simulink library "neuromorphic_blocks"  (R2022a)
settings: Solver=VariableStepAuto  StartTime=0.0  StopTime=10.0  RelTol=1e-3
libraries: $bdroot x31, simulink x7
(part 1 of 2)
settings Model: Creator=chris  LastModifiedBy=chris

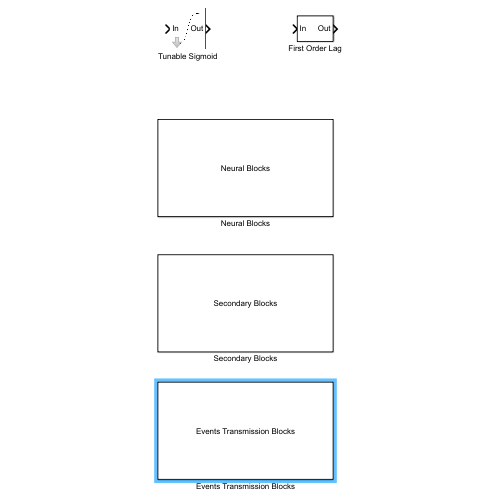
[thumbnail: Simulink's stored preview of the top-level diagram]
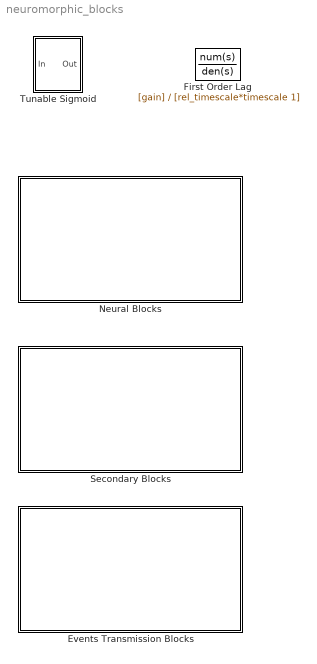
== system neuromorphic_blocks ==
  Events Transmission Blocks : Subsystem
      mask Display: disp('Events Transmission Blocks');
  First Order Lag : TransferFcn  Numerator=[gain]  Denominator=[rel_timescale*timescale 1]  mask(First Order Lag){gain=1, timescale=0.004, rel_timescale=1}
      mask help: Wrapper around Low-Pass Filter block of simulink to make it consistent with other blocks in the toolbox.
      mask DialogControl gain_text Prompt: Gain
      mask DialogControl timescale_text Prompt: Timescale
      mask DialogControl rel_timescale_text Prompt: Relative Timescale
      mask Display:
      | port_label('output', 1, 'Out');
      | port_label('input', 1, 'In');
  Neural Blocks : Subsystem
      mask Display: disp('Neural Blocks');
  Secondary Blocks : Subsystem
      mask Display: disp('Secondary Blocks');
  Tunable Sigmoid : Subsystem  mask(Tunable Sigmoid){nonlinearity_type=Sigmoid, gain_source=Internal, gain=0, bias=0, slope=1}
      mask prompts: gain_source "Source"; gain "Value"; bias "Value"; slope "Value"
      mask help:
      | Sigmoid where gain can be set by external input.
      | The block can be set in Tanh or Sigmoid mode.
      mask init:
      | mask  = Simulink.Mask.get(gcb);
      | 
      |     %type_chosen = mask.getParameter('nonlinearity_type').Value;
      |     %set_param([gcb '/VSNK' ],'LabelModeActiveChoice', type_chosen);
      |     %set_param([gcb '/VSRC' ],'LabelModeActiveChoice', type_chosen);
      |     %disp(type_chosen)
      | 
      |     switch mask.getParameter('nonlinearity_type').Value
      |         case 'Sigmoid'
      |             set_param([gcb '/VSNK' ],'LabelModeActiveChoice', 'Sigmoid');
      |             set_param([gcb '/VSRC' ],'LabelModeActiveChoice', 'Sigmoid');
      |         case 'Tanh'
      |             set_param([gcb '/VSNK' ],'LabelModeActiveChoice', 'Tanh');
      |             set_param([gcb '/VSRC' ],'LabelModeActiveChoice', 'Tanh');
      |     end
      | 
      | 
      |     type = {get_param([gcb '/gain'],'BlockType')};
      |     switch mask.getParameter('gain_source').Value
      |         case 'Internal'
      |             if ismember(type, {'Inport'})
      |                 replace_block([gcb '/gain'], 'Inport', 'Constant', 'noprompt');
      |             end
      |             set_param([gcb '/gain'],'Value','gain');
      |         case 'External'
      |             if ismember(type, {'Constant'})
      |                 replace_block([gcb '/gain'], 'Constant', 'Inport', 'noprompt');
      |             end
      |     end
      mask TypeOptions nonlinearity_type: Sigmoid | Tanh
      mask TypeOptions gain_source: Internal | External
      mask Callback gain_source:
      | mask  = Simulink.Mask.get(gcb);
      |     switch mask.getParameter('gain_source').Value
      |         case 'Internal'
      |             mask.getParameter('gain').Enabled = 'on';
      |         case 'External'
      |             mask.getParameter('gain').Enabled = 'off';
      |     end
      mask DialogControl type_text Prompt: Type
      mask DialogControl gain_text Prompt: Gain
      mask DialogControl bias_text Prompt: Bias
      mask DialogControl slope_text Prompt: Slope
      mask Display:
      | mask  = Simulink.Mask.get(gcb);
      | [gain, gain_converted] = str2num(mask.getParameter('gain').Value);
      | [slope, slope_converted] = str2num(mask.getParameter('slope').Value);
      | 
      | if strcmp(mask.getParameter('gain_source').Value,'Internal') ...
      |    && gain_converted && slope_converted && gain*slope < 0
      |     image('icons/tanh_reversed.jpg');
      | else
      |     image('icons/tanh.jpg');
      | end
      | 
      | 
      | port_label('output', 1, 'Out');
      | 
      | simBlockH = get_param(gcb, 'Handle');
      | portH = find_system(simBlockH, 'LookUnderMasks', 'on', 'FollowLinks', 'on', 'SearchDepth', 1, 'BlockType', 'Inport');
      | portNames = cellstr(get_param(portH, 'Name'));
      | portNum = cellstr(get_param(portH, 'Port'));
      | for i = 1:length(portNames)
      |     if ~isempty(portNames{i})
      |         num = str2num(['uint8(' portNum{i} ')']);
      |         port_label('input', num, portNames{i});
      |     end
      | end

== system neuromorphic_blocks/Events Transmission Blocks ==
  Continuous to Event : Subsystem  mask(Continuous to Event){thresh=0}
      mask prompts: thresh "Value"
      mask DialogControl thresh_text Prompt: Threshold
      mask Display:
      | port_label('output', 1, 'Out');
      | port_label('input', 1, 'In');
  Event Loss : Subsystem  mask(Event Loss){loss_prob=0, seed=-1, seed_mem=randi([0, 100000])}
      mask prompts: loss_prob "Value"; seed "Value"
      mask init:
      | mask  = Simulink.Mask.get(gcb);
      |     switch mask.getParameter('seed').Value
      |         case '-1'
      |             mask.getParameter('seed_mem').Value = 'randi([0, 100000])';
      |         otherwise
      |             mask.getParameter('seed_mem').Value = mask.getParameter('seed').Value;
      |     end
      mask DialogControl loss_prob_text Prompt: Probability of lost event
      mask DialogControl seed_text Prompt: Seed (-1 for random seed)
      mask Display:
      | port_label('output', 1, 'Out');
      | port_label('input', 1, 'In');
  Event to Continuous : Subsystem  mask(Event to Continuous){gain=0}
      mask prompts: gain "Value"
      mask DialogControl gain_text Prompt: Event gain
      mask Display:
      | port_label('output', 1, 'Out');
      | port_label('input', 1, 'In');
  Event to Fixed Width Pulse : Subsystem  mask(Event to Fixed Width Pulse){pulse_width=0}
      mask prompts: pulse_width "Value"
      mask DialogControl pulse_width_text Prompt: Pulse Width
      mask Display:
      | port_label('output', 1, 'Out');
      | port_label('input', 1, 'In');

== system neuromorphic_blocks/Neural Blocks ==
  Modulatory Synapse : Subsystem  mask(Modulatory Synapse){base_val=0, gsyn_pos_source=Internal, gsyn_pos=0, gsyn_neg_source=Internal, gsyn_neg=0, timescale=0.004, rel_timescale=1000, input=Events, dsyn_pos=0, dsyn_neg=0, msyn_pos=1, msyn_neg=1}
      mask prompts: base_val "Value"; gsyn_pos_source "Source"; gsyn_pos "Value"; gsyn_neg_source "Source"; gsyn_neg "Value"; timescale "Value"; rel_timescale "Value"; dsyn_pos "Value"; dsyn_neg "Value"; msyn_pos "Value"; msyn_neg "Value"
      mask init:
      | mask  = Simulink.Mask.get(gcb);
      | 
      |     switch mask.getParameter('input').Value
      |         case 'Events'
      |             set_param([gcb '/VSNK_pos'],'LabelModeActiveChoice', 'Events');
      |             set_param([gcb '/VSRC_pos'],'LabelModeActiveChoice', 'Events');
      |             set_param([gcb '/VSNK_neg'],'LabelModeActiveChoice', 'Events');
      |             set_param([gcb '/VSRC_neg'],'LabelModeActiveChoice', 'Events');
      |             %mask.getPortConstraint('in_main_type').Rule.DataType = {'boolean'};
      |             try
      |                 set_param([gcb '/V+'], 'Name', 'Ev+');
      |                 set_param([gcb '/V-'], 'Name', 'Ev-');
      |             catch E
      |             end
      |         case 'Voltage'
      |             set_param([gcb '/VSNK_pos'],'LabelModeActiveChoice', 'Voltage');
      |             set_param([gcb '/VSRC_pos'],'LabelModeActiveChoice', 'Voltage');
      |             set_param([gcb '/VSNK_neg'],'LabelModeActiveChoice', 'Voltage');
      |             set_param([gcb '/VSRC_neg'],'LabelModeActiveChoice', 'Voltage');
      |             %mask.getPortConstraint('in_main_type').Rule.DataType = {'double'; 'single'; 'int8'; 'uint8'; 'int16'; 'uint16'; 'int32'; 'uint32'};
      |             try
      |                 set_param([gcb '/Ev+'], 'Name', 'V+');
      |                 set_param([gcb '/Ev-'], 'Name', 'V-');
      |             catch E
      |             end
      |     end
      | 
      |     switch mask.getParameter('gsyn_pos_source').Value
      |         case 'Internal'
      |             replace_block([gcb '/gsyn_pos'], 'Inport', 'Constant', 'noprompt');
      |             set_param([gcb '/gsyn_pos'],'Value','gsyn_pos');
      |             if strcmp('0', mask.getParameter(['gsyn_pos']).Value)
      |                 set_param([gcb '/Isyn_pos'],'Commented','on')
      |             else
      |                 set_param([gcb '/Isyn_pos'],'Commented','off')
      |             end
      |         case 'External'
      |             set_param([gcb '/Isyn_pos'],'Commented','on')
      |             replace_block([gcb '/gsyn_pos'], 'Constant', 'Inport', 'noprompt');
      |     end
      | 
      |     switch mask.getParameter('gsyn_neg_source').Value
      |         case 'Internal'
      |             replace_block([gcb '/gsyn_neg'], 'Inport', 'Constant', 'noprompt');
      |             set_param([gcb '/gsyn_neg'],'Value','gsyn_neg');
      |             if strcmp('0', mask.getParameter(['gsyn_neg']).Value)
      |                 set_param([gcb '/Isyn_neg'],'Commented','on')
      |             else
      |                 set_param([gcb '/Isyn_neg'],'Commented','off')
      |             end
      |         case 'External'
      |             set_param([gcb '/Isyn_neg'],'Commented','on')
      |             replace_block([gcb '/gsyn_neg'], 'Constant', 'Inport', 'noprompt');
      |     end
      mask TypeOptions gsyn_pos_source: Internal | External
      mask Callback gsyn_pos_source:
      | mask  = Simulink.Mask.get(gcb);
      |     switch mask.getParameter('gsyn_pos_source').Value
      |         case 'Internal'
      |             mask.getParameter('gsyn_pos').Enabled = 'on';
      |         case 'External'
      |             mask.getParameter('gsyn_pos').Enabled = 'off';
      |     end
      mask TypeOptions gsyn_neg_source: Internal | External
      mask Callback gsyn_neg_source:
      | mask  = Simulink.Mask.get(gcb);
      |     switch mask.getParameter('gsyn_neg_source').Value
      |         case 'Internal'
      |             mask.getParameter('gsyn_neg').Enabled = 'on';
      |         case 'External'
      |             mask.getParameter('gsyn_neg').Enabled = 'off';
      |     end
      mask TypeOptions input: Events | Voltage
      mask Callback input:
      | mask = Simulink.Mask.get(gcb);
      |     switch mask.getParameter('input').Value
      |         case 'Events'
      |             mask.getParameter('dsyn_pos').Enabled = 'off';
      |             mask.getParameter('dsyn_pos').Visible = 'off';
      |             mask.getDialogControl('dsyn_pos_text').Enabled = 'off';
      |             mask.getDialogControl('dsyn_pos_text').Visible = 'off';
      |             mask.getParameter('dsyn_neg').Enabled = 'off';
      |             mask.getParameter('dsyn_neg').Visible = 'off';
      |             mask.getDialogControl('dsyn_neg_text').Enabled = 'off';
      |             mask.getDialogControl('dsyn_neg_text').Visible = 'off';
      |             mask.getParameter('msyn_pos').Enabled = 'off';
      |             mask.getParameter('msyn_pos').Visible = 'off';
      |             mask.getDialogControl('msyn_pos_text').Enabled = 'off';
      |             mask.getDialogControl('msyn_pos_text').Visible = 'off';
      |             mask.getParameter('msyn_neg').Enabled = 'off';
      |             mask.getParameter('msyn_neg').Visible = 'off';
      |             mask.getDialogControl('msyn_neg_text').Enabled = 'off';
      |             mask.getDialogControl('msyn_neg_text').Visible = 'off';
      |         case 'Voltage'
      |             mask.getParameter('dsyn_pos').Enabled = 'on';
      |             mask.getParameter('dsyn_pos').Visible = 'on';
      |             mask.getDialogControl('dsyn_pos_text').Enabled = 'on';
      |             mask.getDialogControl('dsyn_pos_text').Visible = 'on';
      |             mask.getParameter('dsyn_neg').Enabled = 'on';
      |             mask.getParameter('dsyn_neg').Visible = 'on';
      |             mask.getDialogControl('dsyn_neg_text').Enabled = 'on';
      |             mask.getDialogControl('dsyn_neg_text').Visible = 'on';
      |             mask.getParameter('msyn_pos').Enabled = 'on';
      |             mask.getParameter('msyn_pos').Visible = 'on';
      |             mask.getDialogControl('msyn_pos_text').Enabled = 'on';
      |             mask.getDialogControl('msyn_pos_text').Visible = 'on';
      |             mask.getParameter('msyn_neg').Enabled = 'on';
      |             mask.getParameter('msyn_neg').Visible = 'on';
      |             mask.getDialogControl('msyn_neg_text').Enabled = 'on';
      |             mask.getDialogControl('msyn_neg_text').Visible = 'on';
      |     end
      mask DialogControl base_val_text Prompt: Start Parameter
      mask DialogControl gsyn_pos_text Prompt: Positive Event Conductance
      mask DialogControl gsyn_neg_text Prompt: Negative Event Conductance
      mask DialogControl timescale_text Prompt: Timescale
      mask DialogControl rel_timescale_text Prompt: Relative Timescale
      mask DialogControl input_text Prompt: Input Type
      mask DialogControl dsyn_pos_text Prompt: Positive Event Bias
      mask DialogControl dsyn_neg_text Prompt: Negative Event Bias
      mask DialogControl msyn_pos_text Prompt: Positive Event Gain
      mask DialogControl msyn_neg_text Prompt: Negative Event Gain
      mask Display:
      | port_label('output', 1, 'param');
      | 
      | simBlockH = get_param(gcb, 'Handle');
      | portH = find_system(simBlockH, 'LookUnderMasks', 'on', 'FollowLinks', 'on', 'SearchDepth', 1, 'BlockType', 'Inport');
      | portNames = cellstr(get_param(portH, 'Name'));
      | portNum = cellstr(get_param(portH, 'Port'));
      | for i = 1:length(portNames)
      |     if ~isempty(portNames{i})
      |         num = str2num(['uint8(' portNum{i} ')']);
      |         port_label('input', num, portNames{i});
      |     end
      | end
  Neuron : Subsystem  mask(Neuron){gfm_source=Internal, gfm=0, gsp_source=Internal, gsp=0, gsm_source=Internal, gsm=0, gup_source=Internal, gup=0, gum_source=Internal, gum=0, dfm=0, dsp=0, dsm=0, dup=0, dum=0, mfm=1, msp=1, msm=1, mup=1, mum=1, timescale=0.004, rel_membrane=0.1, rel_fast=0.1, rel_slow=4, rel_ultraslow=200, Iapp_base=0, V0=0, tresh=0, output=Events}
      mask prompts: gfm_source "Source"; gfm "Value"; gsp_source "Source"; gsp "Value"; gsm_source "Source"; gsm "Value"; gup_source "Source"; gup "Value"; gum_source "Source"; gum "Value"; dfm "Value"; dsp "Value"; dsm "Value"; dup "Value"; dum "Value"; mfm "Value"; msp "Value"; msm "Value"; mup "Value"; mum "Value"; timescale "Value"; rel_membrane "Value"; rel_fast "Value"; rel_slow "Value"; rel_ultraslow "Value"; Iapp_base "Value"; V0 "Value"; tresh "Value"
      mask help:
      | Block simulating a simplified neuron model (L. Ribar and R. Sepulchre 2019).
      | The conductances can either be set or given as external inputs for neuromodulation.
      mask init:
      | mask  = Simulink.Mask.get(gcb);
      |     
      |     suffix_list = {'fm','sp','sm','up','um'};
      |     
      |     for suffix_cell = suffix_list
      |         suffix = suffix_cell{1};
      |         %block = find_system(gcb, 'LookUnderMasks', 'on', ...
      |         %                        'FollowLinks', 'on', 'Name', ['g' suffix]);
      |         %if isempty(block) 
      |             % Something is very wrong, recreate block
      |         %    add_block('built-in/Constant', [gcb '/g' suffix])
      |         %    h = get_param([gcb '/I' suffix],'LineHandles');
      |         %    if h.Inport(2) > 0
      |         %        delete_line(h.Inport(2)); 
      |         %    end 
      |         %    add_line(gcb,['g' suffix '/1'],['I' suffix '/2']);
      |         %end
      |     
      |         type = get_param([gcb '/g' suffix],'BlockType');
      |         switch mask.getParameter(['g' suffix '_source']).Value
      |             case 'Internal'
      |                 switch type
      |                     case 'Inport'
      |                         replace_block([gcb '/g' suffix], 'Inport', 'Constant', 'noprompt');
      |                         set_param([gcb '/g' suffix],'Value',['g' suffix]);
      |                 end
      |                 if strcmp('0', mask.getParameter(['g' suffix ]).Value)
      |                     set_param([gcb '/I' suffix],'Commented','on')
      |                     set_param([gcb '/g' suffix],'Commented','on')
      |                     set_param([gcb '/I' suffix '_sub'],'Commented','on')
      |                 else
      |                     set_param([gcb '/I' suffix],'Commented','off')
      |                     set_param([gcb '/g' suffix],'Commented','off')
      |                     set_param([gcb '/I' suffix '_sub'],'Commented','off')
      |                 end
      |             case 'External'
      |                 switch type
      |                     case 'Constant'
      |                         replace_block([gcb '/g' suffix], 'Constant', 'Inport', 'noprompt');
      |                 end
      |                 set_param([gcb '/I' suffix],'Commented','off')
      |                 set_param([gcb '/g' suffix],'Commented','off')
      |                 set_param([gcb '/I' suffix '_sub'],'Commented','off')
      |         end
      |     end
      | 
      |     type_V = get_param([gcb '/V'],'BlockType');
      |     type_Ev = get_param([gcb '/Ev'],'BlockType');
      |     switch mask.getParameter('output').Value
      |         case 'Events'
      |             switch type_V
      |                 case 'Outport'
      |                     replace_block([gcb '/V'], 'Outport', 'Terminator', 'noprompt')
      |             end
      |             switch type_Ev
      |                 case 'Terminator'
      |                     replace_block([gcb '/Ev'], 'Terminator', 'Outport', 'noprompt')
      |             end
      |             set_param([gcb '/V_to_Ev'],'Commented','off')
      |         case 'Voltage'
      |             switch type_V
      |                 case 'Terminator'
      |                     replace_block([gcb '/V'], 'Terminator', 'Outport', 'noprompt')
      |             end
      |             switch type_Ev
      |                 case 'Outport'
      |                     replace_block([gcb '/Ev'], 'Outport', 'Terminator', 'noprompt')
      |             end
      |             set_param([gcb '/V_to_Ev'],'Commented','on')
      |         case 'Both'
      |             switch type_Ev
      |                 case 'Terminator'
      |                     switch type_V
      |                         case 'Outport'
      |                             replace_block([gcb '/V'], 'Outport', 'Terminator', 'noprompt')
      |                             type_V = 'Terminator';
      |                     end
      |                     replace_block([gcb '/Ev'], 'Terminator', 'Outport', 'noprompt')
      |             end
      |             switch type_V
      |                 case 'Terminator'
      |                     replace_block([gcb '/V'], 'Terminator', 'Outport', 'noprompt')
      |             end
      |             set_param([gcb '/V_to_Ev'],'Commented','off')
      |     end
      mask TypeOptions gfm_source: Internal | External
      mask Callback gfm_source:
      | source_name = 'gfm_source';
      |     tgt_name = 'gfm';
      |     mask  = Simulink.Mask.get(gcb);
      |     switch mask.getParameter(source_name).Value
      |         case 'Internal'
      |             mask.getParameter(tgt_name).Enabled = 'on';
      |         case 'External'
      |             mask.getParameter(tgt_name).Enabled = 'off';
      |     end
      mask TypeOptions gsp_source: Internal | External
      mask Callback gsp_source:
      | source_name = 'gsp_source';
      |     tgt_name = 'gsp';
      |     mask  = Simulink.Mask.get(gcb);
      |     switch mask.getParameter(source_name).Value
      |         case 'Internal'
      |             mask.getParameter(tgt_name).Enabled = 'on';
      |         case 'External'
      |             mask.getParameter(tgt_name).Enabled = 'off';
      |     end
      mask TypeOptions gsm_source: Internal | External
      mask Callback gsm_source:
      | source_name = 'gsm_source';
      |     tgt_name = 'gsm';
      |     mask  = Simulink.Mask.get(gcb);
      |     switch mask.getParameter(source_name).Value
      |         case 'Internal'
      |             mask.getParameter(tgt_name).Enabled = 'on';
      |         case 'External'
      |             mask.getParameter(tgt_name).Enabled = 'off';
      |     end
      mask TypeOptions gup_source: Internal | External
      mask Callback gup_source:
      | source_name = 'gup_source';
      |     tgt_name = 'gup';
      |     mask  = Simulink.Mask.get(gcb);
      |     switch mask.getParameter(source_name).Value
      |         case 'Internal'
      |             mask.getParameter(tgt_name).Enabled = 'on';
      |         case 'External'
      |             mask.getParameter(tgt_name).Enabled = 'off';
      |     end
      mask TypeOptions gum_source: Internal | External
      mask Callback gum_source:
      | source_name = 'gum_source';
      |     tgt_name = 'gum';
      |     mask  = Simulink.Mask.get(gcb);
      |     switch mask.getParameter(source_name).Value
      |         case 'Internal'
      |             mask.getParameter(tgt_name).Enabled = 'on';
      |         case 'External'
      |             mask.getParameter(tgt_name).Enabled = 'off';
      |     end
      mask TypeOptions output: Events | Voltage | Both
      mask Callback output:
      | source_name = 'output';
      |     tgt_name = 'tresh';
      |     mask  = Simulink.Mask.get(gcb);
      |     switch mask.getParameter(source_name).Value
      |         case 'Voltage'
      |             mask.getParameter(tgt_name).Enabled = 'off';
      |         otherwise
      |             mask.getParameter(tgt_name).Enabled = 'on';
      |     end
      mask DialogControl ConductancesContainer Prompt: Conductances
      mask DialogControl gfm_text Prompt: Fast Negative Conductance (gfm)
      mask DialogControl gsp_text Prompt: Slow Positive Conductance (gsp)
      mask DialogControl gsm_text Prompt: Slow Negative Conductance (gsm)
      mask DialogControl gup_text Prompt: Ultra-Slow Positive Conductance (gup)
      mask DialogControl gum_text Prompt: Ultra-Slow Negative Conductance (gum)
      mask DialogControl BiasesContainer Prompt: Biases
      mask DialogControl dfm_text Prompt: Fast Negative Bias (dfm)
      mask DialogControl dsp_text Prompt: Slow Positive Bias (dsp)
      mask DialogControl dsm_text Prompt: Slow Negative Bias (dsm)
      mask DialogControl dup_text Prompt: Ultra-Slow Positive Bias (gup)
      mask DialogControl dum_text Prompt: Ultra-Slow Negative Bias (gum)
      mask DialogControl SlopesContainer Prompt: Slopes
      mask DialogControl mfm_text Prompt: Fast Negative Slope (mfm)
      mask DialogControl msp_text Prompt: Slow Positive Slope (msp)
      mask DialogControl msm_text Prompt: Slow Negative Slope (msm)
      mask DialogControl mup_text Prompt: Ultra-Slow Positive Slope (mup)
      mask DialogControl mum_text Prompt: Ultra-Slow Negative Slope (mum)
      mask DialogControl TimescalesContainer Prompt: Timescales
      mask DialogControl timescale_text Prompt: Timescale
      mask DialogControl memb_text Prompt: Relative Membrane Timescale
      mask DialogControl fast_text Prompt: Relative Fast Timescale
      mask DialogControl slow_text Prompt: Relative Slow Timescale
      mask DialogControl ultraslow_text Prompt: Relative Ultra-Slow Timescale
      mask DialogControl OtherContainer Prompt: Other
      mask DialogControl Iapp_text Prompt: Base Applied Current
      mask DialogControl V0_text Prompt: Base Voltage
      mask DialogControl tresh_text Prompt: Event Threshold
      mask DialogControl output_text Prompt: Output
      mask Display:
      | pos = get_param(gcb, 'Position');
      | width = pos(3) - pos(1);
      | height = pos(4) - pos(2);
      | 
      | image('icons/neuron.jpg');
      | 
      | simBlockH = get_param(gcb, 'Handle');
      | 
      | 
      | portH = find_system(simBlockH, 'LookUnderMasks', 'on', 'FollowLinks', 'on', 'SearchDepth', 1, 'BlockType', 'Inport');
      | portNames = cellstr(get_param(portH, 'Name'));
      | portNum = cellstr(get_param(portH, 'Port'));
      | for i = 1:length(portNames)
      |     if ~isempty(portNames{i})
      |         num = str2num(['uint8(' portNum{i} ')']);
      |         port_label('input', num, portNames{i});
      |     end
      | end
      | 
      | portH = find_system(simBlockH, 'LookUnderMasks', 'on', 'FollowLinks', 'on', 'SearchDepth', 1, 'BlockType', 'Outport');
      | portNames = cellstr(get_param(portH, 'Name'));
      | portNum = cellstr(get_param(portH, 'Port'));
      | for i = 1:length(portNames)
      |     if ~isempty(portNames{i})
      |         num = str2num(['uint8(' portNum{i} ')']);
      |         port_label('output', num, portNames{i});
      |     end
      | end
  Synapse with Depression : Subsystem  mask(Synapse with Depression){gsyn_source=Internal, gsyn=0, dsyn=0, msyn=1, dsyn_dep=0, msyn_dep=1, timescale=0.004, rel_timescale=100, input=Events, gsyn_in=0, dsyn_in=0, msyn_in=1}
      mask prompts: gsyn_source "Source"; gsyn "Value"; dsyn "Value"; msyn "Value"; dsyn_dep "Value"; msyn_dep "Value"; timescale "Value"; rel_timescale "Value"; gsyn_in "Value"; dsyn_in "Value"; msyn_in "Value"
      mask help: Synapse that lets through the first spikes
      mask init:
      | mask  = Simulink.Mask.get(gcb);
      |     %block = find_system(gcb, 'LookUnderMasks', 'on', ...
      |     %                    'FollowLinks', 'on', 'Name', 'gsyn');
      |     %if isempty(block) 
      |         % Something is very wrong, recreate block
      |     %    add_block('built-in/Constant', [gcb '/gsyn'])
      |     %    h = get_param([gcb '/Sigmoid'],'LineHandles');
      |     %    if h.Inport(2) > 0
      |     %        delete_line(h.Inport(2)); 
      |     %    end 
      |     %    add_line(gcb,'gsyn/1','Sigmoid/2');
      |     %    h = get_param([gcb '/Out Depression Sigmoid'],'LineHandles');
      |     %    if h.Inport(2) > 0
      |     %        delete_line(h.Inport(2)); 
      |     %    end 
      |     %    add_line(gcb,'gsyn/1','Out Depression Sigmoid/2');
      |     %end
      | 
      |     switch mask.getParameter('input').Value
      |         case 'Events'
      |             set_param([gcb '/VSNK' ],'LabelModeActiveChoice', 'Events');
      |             set_param([gcb '/VSRC' ],'LabelModeActiveChoice', 'Events');
      |             %mask.getPortConstraint('in_main_type').Rule.DataType = {'boolean'};
      |             try
      |                 set_param([gcb '/V'], 'Name', 'Ev');
      |             catch E
      |             end
      |         case 'Voltage'
      |             set_param([gcb '/VSNK' ],'LabelModeActiveChoice', 'Voltage');
      |             set_param([gcb '/VSRC' ],'LabelModeActiveChoice', 'Voltage');
      |             %mask.getPortConstraint('in_main_type').Rule.DataType = {'double'; 'single'; 'int8'; 'uint8'; 'int16'; 'uint16'; 'int32'; 'uint32'};
      |             try
      |                 set_param([gcb '/Ev'], 'Name', 'V');
      |             catch E
      |             end
      |     end
      | 
      |     switch mask.getParameter('gsyn_source').Value
      |         case 'Internal'
      |             replace_block([gcb '/gsyn'], 'Inport', 'Constant', 'noprompt');
      |             set_param([gcb '/gsyn'],'Value','gsyn');
      |         case 'External'
      |             replace_block([gcb '/gsyn'], 'Constant', 'Inport', 'noprompt');
      |     end
      mask TypeOptions gsyn_source: Internal | External
      mask Callback gsyn_source:
      | mask  = Simulink.Mask.get(gcb);
      |     switch mask.getParameter('gsyn_source').Value
      |         case 'Internal'
      |             mask.getParameter('gsyn').Enabled = 'on';
      |         case 'External'
      |             mask.getParameter('gsyn').Enabled = 'off';
      |     end
      mask TypeOptions input: Events | Voltage
      mask Callback input:
      | mask = Simulink.Mask.get(gcb);
      |     switch mask.getParameter('input').Value
      |         case 'Events'
      |             mask.getParameter('gsyn_in').Enabled = 'off';
      |             mask.getParameter('gsyn_in').Visible = 'off';
      |             mask.getDialogControl('gsyn_in_text').Enabled = 'off';
      |             mask.getDialogControl('gsyn_in_text').Visible = 'off';
      |             mask.getParameter('dsyn_in').Enabled = 'off';
      |             mask.getParameter('dsyn_in').Visible = 'off';
      |             mask.getDialogControl('dsyn_in_text').Enabled = 'off';
      |             mask.getDialogControl('dsyn_in_text').Visible = 'off';
      |             mask.getParameter('msyn_in').Enabled = 'off';
      |             mask.getParameter('msyn_in').Visible = 'off';
      |             mask.getDialogControl('msyn_in_text').Enabled = 'off';
      |             mask.getDialogControl('msyn_in_text').Visible = 'off';
      |         case 'Voltage'
      |             mask.getParameter('gsyn_in').Enabled = 'on';
      |             mask.getParameter('gsyn_in').Visible = 'on';
      |             mask.getDialogControl('gsyn_in_text').Enabled = 'on';
      |             mask.getDialogControl('gsyn_in_text').Visible = 'on';
      |             mask.getParameter('dsyn_in').Enabled = 'on';
      |             mask.getParameter('dsyn_in').Visible = 'on';
      |             mask.getDialogControl('dsyn_in_text').Enabled = 'on';
      |             mask.getDialogControl('dsyn_in_text').Visible = 'on';
      |             mask.getParameter('msyn_in').Enabled = 'on';
      |             mask.getParameter('msyn_in').Visible = 'on';
      |             mask.getDialogControl('msyn_in_text').Enabled = 'on';
      |             mask.getDialogControl('msyn_in_text').Visible = 'on';
      |     end
      mask DialogControl gsyn_text Prompt: Conductance (gsyn)
      mask DialogControl dsyn_text Prompt: Bias (dsyn)
      mask DialogControl msyn_text Prompt: Slope (msyn)
      mask DialogControl dsyn_dep_text Prompt: Depression Bias (dsyn_dep)
      mask DialogControl msyn_dep_text Prompt: Depression Slope (msyn_dep)
      mask DialogControl timescale_text Prompt: Timescale
      mask DialogControl rel_timescale_text Prompt: Relative Timescale
      mask DialogControl input_text Prompt: Input Type
      mask DialogControl gsyn_in_text Prompt: Input Conductance (gsyn_in)
      mask DialogControl dsyn_in_text Prompt: Inout Bias (dsyn_in)
      mask DialogControl msyn_in_text Prompt: Input Slope (msyn_in)
      mask Display:
      | mask  = Simulink.Mask.get(gcb);
      | [gsyn, gsyn_converted] = str2num(mask.getParameter('gsyn').Value);
      | 
      | if strcmp(mask.getParameter('gsyn_source').Value,'Internal') ...
      |    && gsyn_converted && gsyn < 0
      |     image('icons/depressing_inhib_syn.jpg');
      | else
      |     image('icons/depressing_excit_syn.jpg');
      | end
      | 
      | port_label('output', 1, 'Isyn');
      | 
      | simBlockH = get_param(gcb, 'Handle');
      | portH = find_system(simBlockH, 'LookUnderMasks', 'on', 'FollowLinks', 'on', 'SearchDepth', 1, 'BlockType', 'Inport');
      | portNames = cellstr(get_param(portH, 'Name'));
      | portNum = cellstr(get_param(portH, 'Port'));
      | for i = 1:length(portNames)
      |     if ~isempty(portNames{i})
      |         num = str2num(['uint8(' portNum{i} ')']);
      |         port_label('input', num, portNames{i});
      |     end
      | end
  Synapse with Facilitation : Subsystem  mask(Synapse with Facilitation){gsyn_source=Internal, gsyn=0, dsyn=0, msyn=1, timescale=0.004, rel_timescale=10, input=Events, gsyn_in=0, dsyn_in=0, msyn_in=1}
      mask prompts: gsyn_source "Source"; gsyn "Value"; dsyn "Value"; msyn "Value"; timescale "Value"; rel_timescale "Value"; gsyn_in "Value"; dsyn_in "Value"; msyn_in "Value"
      mask help: Synapse that transmit well long packets of spikes
      mask init:
      | mask  = Simulink.Mask.get(gcb);
      |     %block = find_system(gcb, 'LookUnderMasks', 'on', ...
      |     %                    'FollowLinks', 'on', 'Name', 'gsyn');
      |     %if isempty(block) 
      |     %    % Something is very wrong, recreate block
      |     %    add_block('built-in/Constant', [gcb '/gsyn'])
      |     %    h = get_param([gcb '/sigmoid'],'LineHandles');
      |     %    if h.Inport(2) > 0
      |     %        delete_line(h.Inport(2)); 
      |     %    end 
      |     %    add_line(gcb,'gsyn/1','sigmoid/2');
      |     %end
      | 
      |     %result = find_system([gcb], 'type', 'Block')
      |     %disp(result)
      |     %disp(gcb)
      | 
      |     switch mask.getParameter('input').Value
      |         case 'Events'
      |             set_param([gcb '/VSNK' ],'LabelModeActiveChoice', 'Events');
      |             set_param([gcb '/VSRC' ],'LabelModeActiveChoice', 'Events');
      |             %mask.getPortConstraint('in_main_type').Rule.DataType = {'boolean'};
      |             try
      |                 set_param([gcb '/V'], 'Name', 'Ev');
      |             catch E
      |             end
      |         case 'Voltage'
      |             set_param([gcb '/VSNK' ],'LabelModeActiveChoice', 'Voltage');
      |             set_param([gcb '/VSRC' ],'LabelModeActiveChoice', 'Voltage');
      |             %mask.getPortConstraint('in_main_type').Rule.DataType = {'double'; 'single'; 'int8'; 'uint8'; 'int16'; 'uint16'; 'int32'; 'uint32'};
      |             try
      |                 set_param([gcb '/Ev'], 'Name', 'V');
      |             catch E
      |             end
      |     end
      | 
      |     switch mask.getParameter('gsyn_source').Value
      |         case 'Internal'
      |             replace_block([gcb '/gsyn'], 'Inport', 'Constant', 'noprompt');
      |             set_param([gcb '/gsyn'],'Value','gsyn');
      |         case 'External'
      |             replace_block([gcb '/gsyn'], 'Constant', 'Inport', 'noprompt');
      |     end
      mask TypeOptions gsyn_source: Internal | External
      mask Callback gsyn_source:
      | mask = Simulink.Mask.get(gcb);
      |     switch mask.getParameter('gsyn_source').Value
      |         case 'Internal'
      |             mask.getParameter('gsyn').Enabled = 'on';
      |         case 'External'
      |             mask.getParameter('gsyn').Enabled = 'off';
      |     end
      mask TypeOptions input: Events | Voltage
      mask Callback input:
      | mask = Simulink.Mask.get(gcb);
      |     switch mask.getParameter('input').Value
      |         case 'Events'
      |             mask.getParameter('gsyn_in').Enabled = 'off';
      |             mask.getParameter('gsyn_in').Visible = 'off';
      |             mask.getDialogControl('gsyn_in_text').Enabled = 'off';
      |             mask.getDialogControl('gsyn_in_text').Visible = 'off';
      |             mask.getParameter('dsyn_in').Enabled = 'off';
      |             mask.getParameter('dsyn_in').Visible = 'off';
      |             mask.getDialogControl('dsyn_in_text').Enabled = 'off';
      |             mask.getDialogControl('dsyn_in_text').Visible = 'off';
      |             mask.getParameter('msyn_in').Enabled = 'off';
      |             mask.getParameter('msyn_in').Visible = 'off';
      |             mask.getDialogControl('msyn_in_text').Enabled = 'off';
      |             mask.getDialogControl('msyn_in_text').Visible = 'off';
      |         case 'Voltage'
      |             mask.getParameter('gsyn_in').Enabled = 'on';
      |             mask.getParameter('gsyn_in').Visible = 'on';
      |             mask.getDialogControl('gsyn_in_text').Enabled = 'on';
      |             mask.getDialogControl('gsyn_in_text').Visible = 'on';
      |             mask.getParameter('dsyn_in').Enabled = 'on';
      |             mask.getParameter('dsyn_in').Visible = 'on';
      |             mask.getDialogControl('dsyn_in_text').Enabled = 'on';
      |             mask.getDialogControl('dsyn_in_text').Visible = 'on';
      |             mask.getParameter('msyn_in').Enabled = 'on';
      |             mask.getParameter('msyn_in').Visible = 'on';
      |             mask.getDialogControl('msyn_in_text').Enabled = 'on';
      |             mask.getDialogControl('msyn_in_text').Visible = 'on';
      |     end
      mask DialogControl gsyn_text Prompt: Conductance (gsyn)
      mask DialogControl dsyn_text Prompt: Bias (dsyn)
      mask DialogControl msyn_text Prompt: Slope (msyn)
      mask DialogControl timescale_text Prompt: Timescale
      mask DialogControl rel_text Prompt: Relative Timescale
      mask DialogControl input_text Prompt: Input Type
      mask DialogControl gsyn_in_text Prompt: Input Conductance (gsyn_in)
      mask DialogControl dsyn_in_text Prompt: Input Bias (dsyn_in)
      mask DialogControl msyn_in_text Prompt: Input Slope (msyn_in)
      mask Display:
      | mask  = Simulink.Mask.get(gcb);
      | [gsyn, gsyn_converted] = str2num(mask.getParameter('gsyn').Value);
      | 
      | if strcmp(mask.getParameter('gsyn_source').Value,'Internal') ...
      |    && gsyn_converted && gsyn < 0
      |     image('icons/facilitating_inhib_syn.jpg');
      | else
      |     image('icons/facilitating_excit_syn.jpg');
      | end
      | 
      | 
      | port_label('output', 1, 'Isyn');
      | 
      | simBlockH = get_param(gcb, 'Handle');
      | portH = find_system(simBlockH, 'LookUnderMasks', 'on', 'FollowLinks', 'on', 'SearchDepth', 1, 'BlockType', 'Inport');
      | portNames = cellstr(get_param(portH, 'Name'));
      | portNum = cellstr(get_param(portH, 'Port'));
      | for i = 1:length(portNames)
      |     if ~isempty(portNames{i})
      |         num = str2num(['uint8(' portNum{i} ')']);
      |         port_label('input', num, portNames{i});
      |     end
      | end
